simulink model "power_KundurTwoAreaSystem"  (R2021b)
settings: Solver=VariableStepAuto  StartTime=0.0  StopTime=20  MaxStep=1/60  RelTol=1e-4
PreLoadFcn:
  | Ts=50e-6;
  | Tctrl=2*Ts;
  | PSSMODEL=1;
model workspace (MAT data in the model file):
  LOL = 0
undefined symbols (not defined in the file or in its folder): D1, Delta
libraries: spsGenericPowerSystemStabilizerLib x8, spsThreePhaseVIMeasurementLib x6, spsLoadFlowBusLib x6, spsThreePhaseParallelRLCLoadLib x4, spsThreePhasePISectionLineLib x4, spsSynchronousMachinepuStandardLib x4, spsExcitationSystemLib x4, spsSteamTurbineandGovernorLib x4, spsThreePhaseSeriesRLCLoadLib x4, spsThreePhaseTransformerTwoWindingsLib x4, spsThreePhaseBreakerLib x2, spsDistributedParametersLineLib x2
(part 2 of 2)

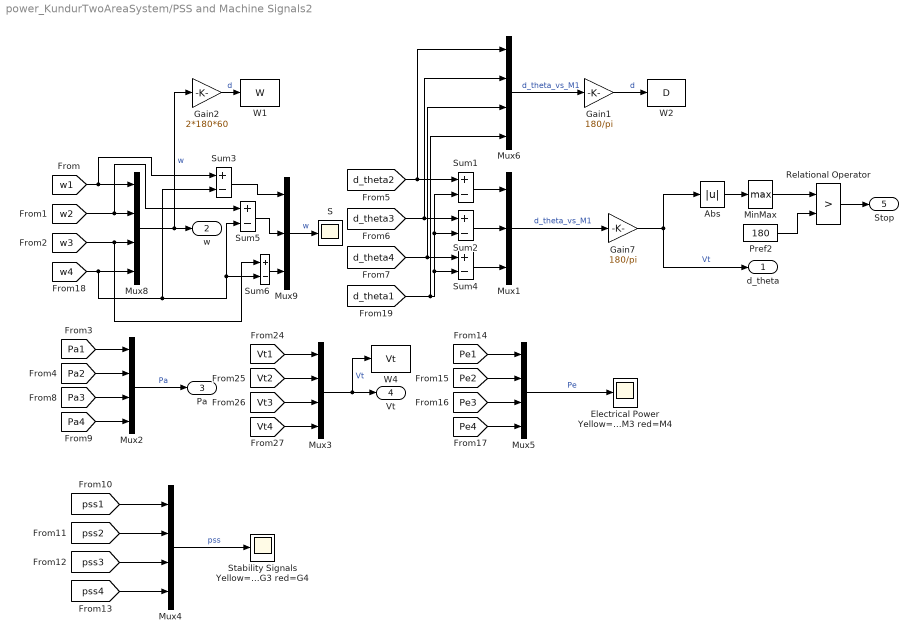
== system power_KundurTwoAreaSystem/PSS and Machine Signals2 ==
  Abs : Abs  SaturateOnIntegerOverflow=on
  "Electrical Power Yellow=M1 mag=M2 cyan=M3 red=M4 " : Scope
  Gain1 : Gain  Gain=180/pi
  Gain2 : Gain  Gain=2*180*60
  Gain7 : Gain  Gain=180/pi
  MinMax : MinMax  Function=max  InputSameDT=on  SaturateOnIntegerOverflow=on
  Mux1 : Mux  Inputs=3
  Mux{2..6,8} (6 alike) : Mux
  Mux9 : Mux  Inputs=3
  Pref2 : Constant  Value=180
  Relational Operator : RelationalOperator  Operator=>  RndMeth=Nearest  InputSameDT=on
  S : Scope
  "Stability Signals Yellow=G1 mag=G2 cyan=G3 red=G4 " : Scope
  Sum{1..6} (6 alike) : Sum  Inputs=+-  InputSameDT=on  SaturateOnIntegerOverflow=on  OutDataTypeStr=Inherit: Same as first input
  W1 : ToWorkspace  VariableName=W  SampleTime=-1
  W2 : ToWorkspace  VariableName=D  SampleTime=-1
  W4 : ToWorkspace  VariableName=Vt  SampleTime=-1
  d_theta : Outport  VectorParamsAs1DForOutWhenUnconnected=off
  w : Outport  Port=2  VectorParamsAs1DForOutWhenUnconnected=off
  Pa : Outport  Port=3  VectorParamsAs1DForOutWhenUnconnected=off
  Vt : Outport  Port=4  VectorParamsAs1DForOutWhenUnconnected=off
  Stop : Outport  Port=5  VectorParamsAs1DForOutWhenUnconnected=off
  wires:
  [Pa1] -> Mux2/1
  Mux4/1 -> "Stability Signals Yellow=G1 mag=G2 cyan=G3 red=G4 "/1  "pss"
  [pss1] -> Mux4/1
  [pss2] -> Mux4/2
  [pss4] -> Mux4/4
  [pss3] -> Mux4/3
  Mux8/1 -> Gain2/1, w/1  "w"
  Relational Operator/1 -> Stop/1
  Mux2/1 -> Pa/1  "Pa"
  [Pa2] -> Mux2/2
  [Pa3] -> Mux2/3
  [Pa4] -> Mux2/4
  [Vt1] -> Mux3/1
  [Vt2] -> Mux3/2
  [Vt3] -> Mux3/3
  [Vt4] -> Mux3/4
  Mux3/1 -> Vt/1, W4/1  "Vt"
  [Pe1] -> Mux5/1
  [Pe2] -> Mux5/2
  [Pe3] -> Mux5/3
  [Pe4] -> Mux5/4
  Mux5/1 -> "Electrical Power Yellow=M1 mag=M2 cyan=M3 red=M4 "/1  "Pe"
  [w1] -> Mux8/1, Sum3/1
  [w2] -> Mux8/2, Sum5/1
  [w3] -> Mux8/3, Sum6/1
  [w4] -> Mux8/4, Sum3/2, Sum6/2, Sum5/2
  Sum3/1 -> Mux9/1
  Sum5/1 -> Mux9/2
  Sum6/1 -> Mux9/3
  Mux1/1 -> Gain7/1  "d_theta_vs_M1"
  Abs/1 -> MinMax/1
  Pref2/1 -> Relational Operator/2
  MinMax/1 -> Relational Operator/1
  [d_theta2] -> Mux6/1, Sum1/1
  Sum1/1 -> Mux1/1
  [d_theta3] -> Mux6/2, Sum2/1
  [d_theta4] -> Mux6/3, Sum4/1
  [d_theta1] -> Mux6/4, Sum4/2, Sum2/2, Sum1/2
  Sum2/1 -> Mux1/2
  Sum4/1 -> Mux1/3
  Mux9/1 -> S/1  "w"
  Gain7/1 -> d_theta/1, Abs/1  "Vt"
  Mux6/1 -> Gain1/1  "d_theta_vs_M1"
  Gain1/1 -> W2/1  "d"
  Gain2/1 -> W1/1  "d"

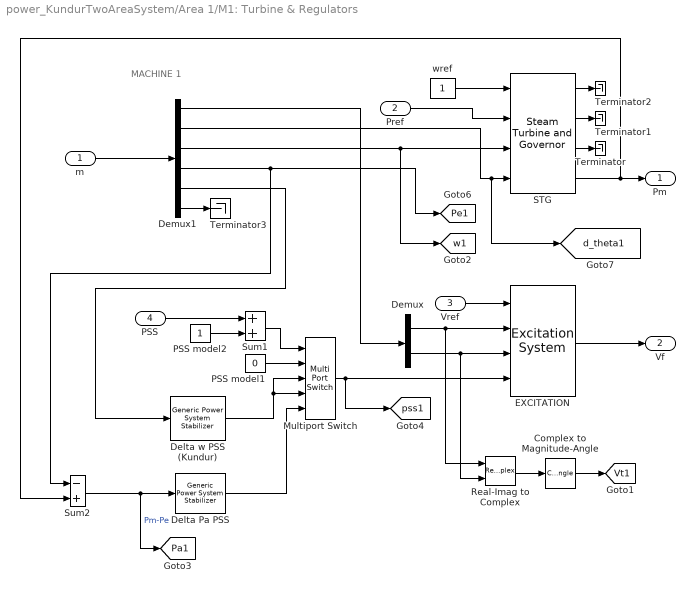
== system power_KundurTwoAreaSystem/Area 1/M1: Turbine & Regulators ==
  note: MACHINE 1
  m : Inport
  Pref : Inport  Port=2
  Vref : Inport  Port=3
  PSS : Inport  Port=4
  Complex to Magnitude-Angle : ComplexToMagnitudeAngle  Output=Magnitude
  Delta Pa PSS : spsGenericPowerSystemStabilizerLib/Generic Power System Stabilizer  Tsensor=15e-3  K=2.5*1.25  Twashout=1  Tleadlag1=[60e-3 1]  Tleadlag2=[0 0]  VSlimits=[-0.15 0.15]  Vinit=0  Plot_On=off  MagdB_On=on  FreqRange=logspace(-2,2,500)
      settings: SourceProductBaseCode=PS
  Delta w PSS (Kundur) : spsGenericPowerSystemStabilizerLib/Generic Power System Stabilizer  Tsensor=15e-3  K=30  Twashout=10  Tleadlag1=[50e-3 20e-3]  Tleadlag2=[3 5.4]  VSlimits=[-0.15 0.15]  Vinit=0  Plot_On=off  MagdB_On=on  FreqRange=logspace(-2,2,500)
      settings: SourceProductBaseCode=PS
  Demux : Demux  Outputs=2
      settings: DisplayOption=none
  Demux1 : Demux  Outputs=[2 1 1 1 1 1]
  EXCITATION : spsExcitationSystemLib/Excitation System  tr=20e-3  reg=[ 200, 0.001 ]  exc=[ 1, 0 ]  tgr=[ 0, 0 ]  damp=[ 0, 0 ]  sat=[ 0, 0 ]  lim=[-12.3 , 12.3, 0 ]  v0=[1,1.83395]
      settings: SourceProductBaseCode=PS
  Multiport Switch : MultiPortSwitch  Inputs=4  InputSameDT=on
  PSS model1 : Constant  Value=0
  PSS model2 : Constant
  Real-Imag to Complex : RealImagToComplex
  STG : spsSteamTurbineandGovernorLib/Steam Turbine and Governor  gentype=Tandem-compound (single mass)  reg1="[ 1  0.05    0 ]"  reg2="[ 0.001  0.15 ]"  reg3="[ -0.1  0.1  0  4.496 ]"  N=3600  turb1="[ 0  10   3.3   0.5   ]"  turb2="[   0   0.36    0.36   0.28   ]"  HA="[ 0.046  1.430  1.465   0.192 ]"  KA="[ 90.44  53.88  64.59   62.94  ]"  DA="[ 0.0115  0.3575  0.3663   0.0137  ]"  ini1=0.7778  ini2=[0.779316,-31.4247]
      settings: SourceProductBaseCode=PS
  Sum1 : Sum  InputSameDT=on  SaturateOnIntegerOverflow=on  OutDataTypeStr=Inherit: Same as first input
  Sum2 : Sum  Inputs=-+  InputSameDT=on  SaturateOnIntegerOverflow=on  OutDataTypeStr=Inherit: Same as first input
  Terminator{,1..3} (4 alike) : Terminator
  wref : Constant
  Pm : Outport  InitialOutput=0  VectorParamsAs1DForOutWhenUnconnected=off
  Vf : Outport  Port=2  InitialOutput=0  VectorParamsAs1DForOutWhenUnconnected=off
  tag scope: Pa1=global, Pe1=global, Vt1=global, d_theta1=global, pss1=global, w1=global
  wires:
  Demux/1 -> Real-Imag to Complex/1, EXCITATION/2
  Demux/2 -> Real-Imag to Complex/2, EXCITATION/3
  wref/1 -> STG/1
  Pref/1 -> STG/2
  m/1 -> Demux1/1
  Vref/1 -> EXCITATION/1
  Real-Imag to Complex/1 -> Complex to Magnitude-Angle/1
  EXCITATION/1 -> Vf/1
  Complex to Magnitude-Angle/1 -> [Vt1]
  Demux1/6 -> Terminator3/1
  PSS model1/1 -> Multiport Switch/2
  Delta w PSS (Kundur)/1 -> Multiport Switch/4, Multiport Switch/3
  Delta Pa PSS/1 -> Multiport Switch/5
  PSS model2/1 -> Sum1/2
  Sum1/1 -> Multiport Switch/1
  PSS/1 -> Sum1/1
  Demux1/1 -> Demux/1
  Demux1/3 -> [w1], STG/3
  Demux1/4 -> Sum2/1, [Pe1]
  Demux1/5 -> Delta w PSS (Kundur)/1
  Sum2/1 -> Delta Pa PSS/1, [Pa1]  "Pm-Pe"
  STG/3 -> Terminator/1
  Demux1/2 -> [d_theta1], STG/4
  STG/4 -> Pm/1, Sum2/2
  STG/2 -> Terminator1/1
  STG/1 -> Terminator2/1
  Multiport Switch/1 -> EXCITATION/4, [pss1]

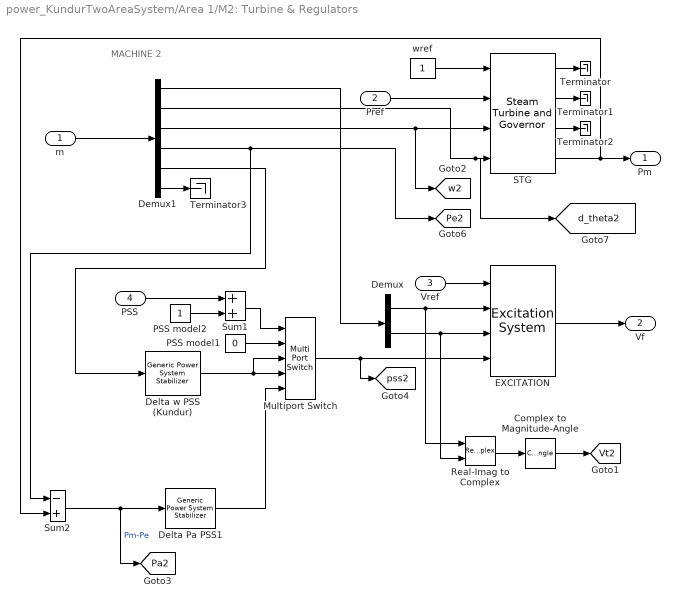
== system power_KundurTwoAreaSystem/Area 1/M2: Turbine & Regulators ==
  note: MACHINE 2
  m : Inport
  Pref : Inport  Port=2
  Vref : Inport  Port=3
  PSS : Inport  Port=4
  Complex to Magnitude-Angle : ComplexToMagnitudeAngle  Output=Magnitude
  Delta Pa PSS1 : spsGenericPowerSystemStabilizerLib/Generic Power System Stabilizer  Tsensor=15e-3  K=2.5*1.25  Twashout=1  Tleadlag1=[60e-3 1]  Tleadlag2=[0 0]  VSlimits=[-0.15 0.15]  Vinit=0  Plot_On=off  MagdB_On=on  FreqRange=logspace(-2,2,500)
      settings: SourceProductBaseCode=PS
  Delta w PSS (Kundur) : spsGenericPowerSystemStabilizerLib/Generic Power System Stabilizer  Tsensor=15e-3  K=30  Twashout=10  Tleadlag1=[50e-3 20e-3]  Tleadlag2=[3 5.4]  VSlimits=[-0.15 0.15]  Vinit=0  Plot_On=off  MagdB_On=on  FreqRange=logspace(-2,2,500)
      settings: SourceProductBaseCode=PS
  Demux : Demux  Outputs=2
      settings: DisplayOption=none
  Demux1 : Demux  Outputs=[2 1 1 1 1 1]
  EXCITATION : spsExcitationSystemLib/Excitation System  tr=20e-3  reg=[ 200, 0.001 ]  exc=[ 1, 0 ]  tgr=[ 0, 0 ]  damp=[ 0, 0 ]  sat=[ 0, 0 ]  lim=[ -12 , 12, 0 ]  v0=[1,1.83395]
      settings: SourceProductBaseCode=PS
  Multiport Switch : MultiPortSwitch  Inputs=4  InputSameDT=on
  PSS model1 : Constant  Value=0
  PSS model2 : Constant
  Real-Imag to Complex : RealImagToComplex
  STG : spsSteamTurbineandGovernorLib/Steam Turbine and Governor  gentype=Tandem-compound (single mass)  reg1="[ 1  0.05    0 ]"  reg2="[ 0.001  0.15 ]"  reg3="[ -0.1  0.1  0  4.496 ]"  N=3600  turb1="[ 0  10   3.3   0.5   ]"  turb2="[   0   0.36    0.36   0.28   ]"  HA="[ 0.046  1.430  1.465   0.192 ]"  KA="[ 90.44  53.88  64.59   62.94  ]"  DA="[ 0.0115  0.3575  0.3663   0.0137  ]"  ini1=0.7777  ini2=[0.779243,-42.8075]
      settings: SourceProductBaseCode=PS
  Sum1 : Sum  InputSameDT=on  SaturateOnIntegerOverflow=on  OutDataTypeStr=Inherit: Same as first input
  Sum2 : Sum  Inputs=-+  InputSameDT=on  SaturateOnIntegerOverflow=on  OutDataTypeStr=Inherit: Same as first input
  Terminator{,1..3} (4 alike) : Terminator
  wref : Constant
  Pm : Outport  InitialOutput=0  VectorParamsAs1DForOutWhenUnconnected=off
  Vf : Outport  Port=2  InitialOutput=0  VectorParamsAs1DForOutWhenUnconnected=off
  tag scope: Pa2=global, Pe2=global, Vt2=global, d_theta2=global, pss2=global, w2=global
  wires:
  Sum2/1 -> Delta Pa PSS1/1, [Pa2]  "Pm-Pe"
  Demux1/5 -> Delta w PSS (Kundur)/1
  Demux1/4 -> Sum2/1, [Pe2]
  Demux1/3 -> [w2], STG/3
  Demux1/1 -> Demux/1
  PSS/1 -> Sum1/1
  Sum1/1 -> Multiport Switch/1
  PSS model2/1 -> Sum1/2
  Delta Pa PSS1/1 -> Multiport Switch/5
  Delta w PSS (Kundur)/1 -> Multiport Switch/4, Multiport Switch/3
  PSS model1/1 -> Multiport Switch/2
  Multiport Switch/1 -> [pss2], EXCITATION/4
  Demux1/6 -> Terminator3/1
  Complex to Magnitude-Angle/1 -> [Vt2]
  EXCITATION/1 -> Vf/1
  Real-Imag to Complex/1 -> Complex to Magnitude-Angle/1
  Vref/1 -> EXCITATION/1
  Pref/1 -> STG/2
  wref/1 -> STG/1
  Demux/2 -> Real-Imag to Complex/2, EXCITATION/3
  Demux/1 -> Real-Imag to Complex/1, EXCITATION/2
  STG/1 -> Terminator/1
  STG/2 -> Terminator1/1
  STG/3 -> Terminator2/1
  STG/4 -> Pm/1, Sum2/2
  Demux1/2 -> [d_theta2], STG/4
  m/1 -> Demux1/1

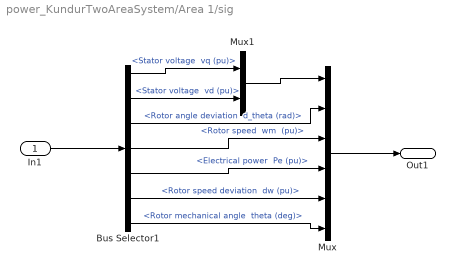
== system power_KundurTwoAreaSystem/Area 1/sig ==
  In1 : Inport
  Bus Selector1 : BusSelector  OutputSignals="dq0 components.Stator voltage  vq (pu),dq0 components.Stator voltage  vd (pu),Mechanical.Rotor angle deviation  d_theta (rad),Mechanical.Rotor speed  wm  (pu),Mechanical.Electrical power  Pe (pu),Mechanical.Rotor speed deviation  dw (pu),Mechanical.Rotor mechanical angle  theta (deg)"
  Mux : Mux  Inputs=6
  Mux1 : Mux  Inputs=2
  Out1 : Outport  VectorParamsAs1DForOutWhenUnconnected=off
  wires:
  Mux/1 -> Out1/1
  In1/1 -> Bus Selector1/1
  Bus Selector1/7 -> Mux/6  "<Rotor mechanical angle  theta (deg)>"
  Bus Selector1/6 -> Mux/5  "<Rotor speed deviation  dw (pu)>"
  Bus Selector1/5 -> Mux/4  "<Electrical power  Pe (pu)>"
  Bus Selector1/4 -> Mux/3  "<Rotor speed  wm  (pu)>"
  Bus Selector1/3 -> Mux/2  "<Rotor angle deviation  d_theta (rad)>"
  Bus Selector1/2 -> Mux1/2  "<Stator voltage  vd (pu)>"
  Bus Selector1/1 -> Mux1/1  "<Stator voltage  vq (pu)>"
  Mux1/1 -> Mux/1

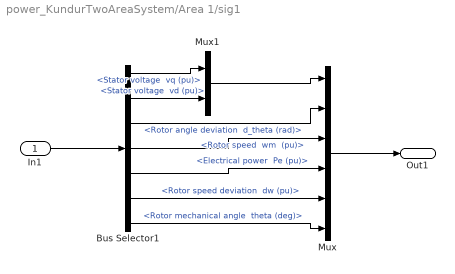
== system power_KundurTwoAreaSystem/Area 1/sig1 ==
  In1 : Inport
  Bus Selector1 : BusSelector  OutputSignals="dq0 components.Stator voltage  vq (pu),dq0 components.Stator voltage  vd (pu),Mechanical.Rotor angle deviation  d_theta (rad),Mechanical.Rotor speed  wm  (pu),Mechanical.Electrical power  Pe (pu),Mechanical.Rotor speed deviation  dw (pu),Mechanical.Rotor mechanical angle  theta (deg)"
  Mux : Mux  Inputs=6
  Mux1 : Mux  Inputs=2
  Out1 : Outport  VectorParamsAs1DForOutWhenUnconnected=off
  wires:
  Mux1/1 -> Mux/1
  Bus Selector1/1 -> Mux1/1  "<Stator voltage  vq (pu)>"
  Bus Selector1/2 -> Mux1/2  "<Stator voltage  vd (pu)>"
  Bus Selector1/3 -> Mux/2  "<Rotor angle deviation  d_theta (rad)>"
  Bus Selector1/4 -> Mux/3  "<Rotor speed  wm  (pu)>"
  Bus Selector1/5 -> Mux/4  "<Electrical power  Pe (pu)>"
  Bus Selector1/6 -> Mux/5  "<Rotor speed deviation  dw (pu)>"
  Bus Selector1/7 -> Mux/6  "<Rotor mechanical angle  theta (deg)>"
  In1/1 -> Bus Selector1/1
  Mux/1 -> Out1/1

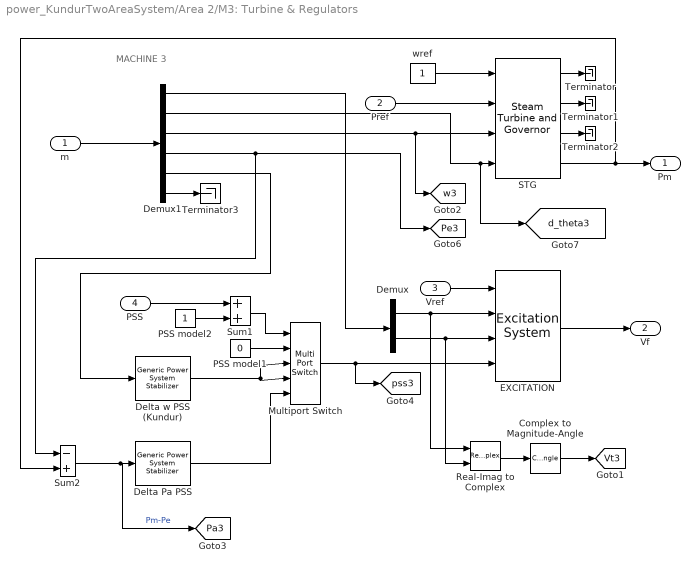
== system power_KundurTwoAreaSystem/Area 2/M3: Turbine & Regulators ==
  note: MACHINE 3
  m : Inport
  Pref : Inport  Port=2
  Vref : Inport  Port=3
  PSS : Inport  Port=4
  Complex to Magnitude-Angle : ComplexToMagnitudeAngle  Output=Magnitude
  Delta Pa PSS : spsGenericPowerSystemStabilizerLib/Generic Power System Stabilizer  Tsensor=15e-3  K=2.5*1.25  Twashout=1  Tleadlag1=[60e-3 1]  Tleadlag2=[0 0]  VSlimits=[-0.15 0.15]  Vinit=0  Plot_On=off  MagdB_On=on  FreqRange=logspace(-2,2,500)
      settings: SourceProductBaseCode=PS
  Delta w PSS (Kundur) : spsGenericPowerSystemStabilizerLib/Generic Power System Stabilizer  Tsensor=15e-3  K=30  Twashout=10  Tleadlag1=[50e-3 20e-3]  Tleadlag2=[3 5.4]  VSlimits=[-0.15 0.15]  Vinit=0  Plot_On=off  MagdB_On=on  FreqRange=logspace(-2,2,500)
      settings: SourceProductBaseCode=PS
  Demux : Demux  Outputs=2
      settings: DisplayOption=none
  Demux1 : Demux  Outputs=[2 1 1 1 1 1]
  EXCITATION : spsExcitationSystemLib/Excitation System  tr=20e-3  reg=[ 200, 0.001 ]  exc=[ 1, 0 ]  tgr=[ 0, 0 ]  damp=[ 0, 0 ]  sat=[ 0, 0 ]  lim=[ -12.3 , 12.3, 0 ]  v0=[1,1.83395]
      settings: SourceProductBaseCode=PS
  Multiport Switch : MultiPortSwitch  Inputs=4  InputSameDT=on
  PSS model1 : Constant  Value=0
  PSS model2 : Constant
  Real-Imag to Complex : RealImagToComplex
  STG : spsSteamTurbineandGovernorLib/Steam Turbine and Governor  gentype=Tandem-compound (single mass)  reg1="[ 1  0.05    0 ]"  reg2="[ 0.001  0.15 ]"  reg3="[ -0.1  0.1  0  4.496 ]"  N=3600  turb1="[ 0  10   3.3   0.5   ]"  turb2="[   0   0.36    0.36   0.28   ]"  HA="[ 0.046  1.430  1.465   0.192 ]"  KA="[ 90.44  53.88  64.59   62.94  ]"  DA="[ 0.0115  0.3575  0.3663   0.0137  ]"  ini1=0.798889  ini2=[0.800505,-56.3243]
      settings: SourceProductBaseCode=PS
  Sum1 : Sum  InputSameDT=on  SaturateOnIntegerOverflow=on  OutDataTypeStr=Inherit: Same as first input
  Sum2 : Sum  Inputs=-+  InputSameDT=on  SaturateOnIntegerOverflow=on  OutDataTypeStr=Inherit: Same as first input
  Terminator{,1..3} (4 alike) : Terminator
  wref : Constant
  Pm : Outport  InitialOutput=0  VectorParamsAs1DForOutWhenUnconnected=off
  Vf : Outport  Port=2  InitialOutput=0  VectorParamsAs1DForOutWhenUnconnected=off
  tag scope: Pa3=global, Pe3=global, Vt3=global, d_theta3=global, pss3=global, w3=global
  wires:
  Sum2/1 -> [Pa3], Delta Pa PSS/1  "Pm-Pe"
  Demux1/5 -> Delta w PSS (Kundur)/1
  Demux1/4 -> Sum2/1, [Pe3]
  Demux1/3 -> [w3], STG/3
  Demux1/1 -> Demux/1
  PSS/1 -> Sum1/1
  Sum1/1 -> Multiport Switch/1
  PSS model2/1 -> Sum1/2
  Delta Pa PSS/1 -> Multiport Switch/5
  Delta w PSS (Kundur)/1 -> Multiport Switch/4, Multiport Switch/3
  PSS model1/1 -> Multiport Switch/2
  Multiport Switch/1 -> [pss3], EXCITATION/4
  Demux1/6 -> Terminator3/1
  Complex to Magnitude-Angle/1 -> [Vt3]
  EXCITATION/1 -> Vf/1
  Real-Imag to Complex/1 -> Complex to Magnitude-Angle/1
  Vref/1 -> EXCITATION/1
  m/1 -> Demux1/1
  Pref/1 -> STG/2
  wref/1 -> STG/1
  Demux/2 -> Real-Imag to Complex/2, EXCITATION/3
  Demux/1 -> Real-Imag to Complex/1, EXCITATION/2
  Demux1/2 -> [d_theta3], STG/4
  STG/1 -> Terminator/1
  STG/2 -> Terminator1/1
  STG/3 -> Terminator2/1
  STG/4 -> Pm/1, Sum2/2

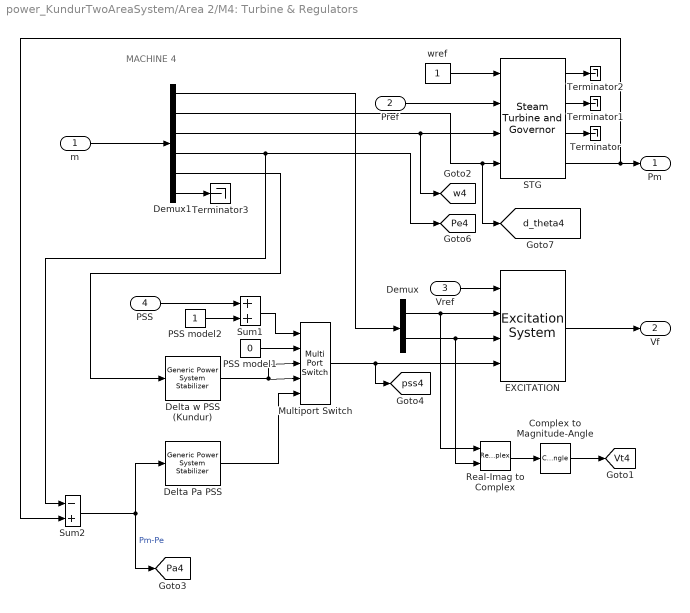
== system power_KundurTwoAreaSystem/Area 2/M4: Turbine & Regulators ==
  note: MACHINE 4
  m : Inport
  Pref : Inport  Port=2
  Vref : Inport  Port=3
  PSS : Inport  Port=4
  Complex to Magnitude-Angle : ComplexToMagnitudeAngle  Output=Magnitude
  "Delta Pa PSS " : spsGenericPowerSystemStabilizerLib/Generic Power System Stabilizer  Tsensor=15e-3  K=2.5*1.25  Twashout=1  Tleadlag1=[60e-3 1]  Tleadlag2=[0 0]  VSlimits=[-0.15 0.15]  Vinit=0  Plot_On=off  MagdB_On=on  FreqRange=logspace(-2,2,500)
      settings: SourceProductBaseCode=PS
  Delta w PSS (Kundur) : spsGenericPowerSystemStabilizerLib/Generic Power System Stabilizer  Tsensor=15e-3  K=30  Twashout=10  Tleadlag1=[50e-3 20e-3]  Tleadlag2=[3 5.4]  VSlimits=[-0.15 0.15]  Vinit=0  Plot_On=off  MagdB_On=on  FreqRange=logspace(-2,2,500)
      settings: SourceProductBaseCode=PS
  Demux : Demux  Outputs=2
      settings: DisplayOption=none
  Demux1 : Demux  Outputs=[2 1 1 1 1 1]
  EXCITATION : spsExcitationSystemLib/Excitation System  tr=20e-3  reg=[ 200, 0.001 ]  exc=[ 1, 0 ]  tgr=[ 0, 0 ]  damp=[ 0, 0 ]  sat=[ 0, 0 ]  lim=[ -12.3 , 12.3, 0 ]  v0=[1,1.83395]
      settings: SourceProductBaseCode=PS
  Multiport Switch : MultiPortSwitch  Inputs=4  InputSameDT=on
  PSS model1 : Constant  Value=0
  PSS model2 : Constant
  Real-Imag to Complex : RealImagToComplex
  STG : spsSteamTurbineandGovernorLib/Steam Turbine and Governor  gentype=Tandem-compound (single mass)  reg1="[ 1  0.05    0 ]"  reg2="[ 0.001  0.15 ]"  reg3="[ -0.1  0.1  0  4.496 ]"  N=3600  turb1="[ 0  10   3.3   0.5   ]"  turb2="[   0   0.36    0.36   0.28   ]"  HA="[ 0.046  1.430  1.465   0.192 ]"  KA="[ 90.44  53.88  64.59   62.94  ]"  DA="[ 0.0115  0.3575  0.3663   0.0137  ]"  ini1=0.7778  ini2=[0.779311,-67.7513]
      settings: SourceProductBaseCode=PS
  Sum1 : Sum  InputSameDT=on  SaturateOnIntegerOverflow=on  OutDataTypeStr=Inherit: Same as first input
  Sum2 : Sum  Inputs=-+  InputSameDT=on  SaturateOnIntegerOverflow=on  OutDataTypeStr=Inherit: Same as first input
  Terminator{,1..3} (4 alike) : Terminator
  wref : Constant
  Pm : Outport  InitialOutput=0  VectorParamsAs1DForOutWhenUnconnected=off
  Vf : Outport  Port=2  InitialOutput=0  VectorParamsAs1DForOutWhenUnconnected=off
  tag scope: Pa4=global, Pe4=global, Vt4=global, d_theta4=global, pss4=global, w4=global
  wires:
  Demux/1 -> Real-Imag to Complex/1, EXCITATION/2
  Demux/2 -> Real-Imag to Complex/2, EXCITATION/3
  STG/4 -> Pm/1, Sum2/2
  wref/1 -> STG/1
  Pref/1 -> STG/2
  m/1 -> Demux1/1
  Vref/1 -> EXCITATION/1
  STG/3 -> Terminator/1
  Real-Imag to Complex/1 -> Complex to Magnitude-Angle/1
  EXCITATION/1 -> Vf/1
  Complex to Magnitude-Angle/1 -> [Vt4]
  Demux1/6 -> Terminator3/1
  Multiport Switch/1 -> EXCITATION/4, [pss4]
  PSS model1/1 -> Multiport Switch/2
  Delta w PSS (Kundur)/1 -> Multiport Switch/4, Multiport Switch/3
  "Delta Pa PSS "/1 -> Multiport Switch/5
  PSS model2/1 -> Sum1/2
  Sum1/1 -> Multiport Switch/1
  PSS/1 -> Sum1/1
  Demux1/1 -> Demux/1
  Demux1/3 -> [w4], STG/3
  Demux1/4 -> Sum2/1, [Pe4]
  Demux1/5 -> Delta w PSS (Kundur)/1
  Sum2/1 -> "Delta Pa PSS "/1, [Pa4]  "Pm-Pe"
  STG/2 -> Terminator1/1
  STG/1 -> Terminator2/1
  Demux1/2 -> [d_theta4], STG/4

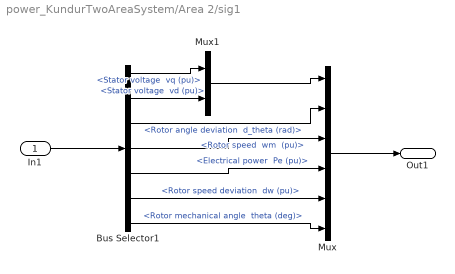
== system power_KundurTwoAreaSystem/Area 2/sig1 ==
  In1 : Inport
  Bus Selector1 : BusSelector  OutputSignals="dq0 components.Stator voltage  vq (pu),dq0 components.Stator voltage  vd (pu),Mechanical.Rotor angle deviation  d_theta (rad),Mechanical.Rotor speed  wm  (pu),Mechanical.Electrical power  Pe (pu),Mechanical.Rotor speed deviation  dw (pu),Mechanical.Rotor mechanical angle  theta (deg)"
  Mux : Mux  Inputs=6
  Mux1 : Mux  Inputs=2
  Out1 : Outport  VectorParamsAs1DForOutWhenUnconnected=off
  wires:
  Mux1/1 -> Mux/1
  Bus Selector1/1 -> Mux1/1  "<Stator voltage  vq (pu)>"
  Bus Selector1/2 -> Mux1/2  "<Stator voltage  vd (pu)>"
  Bus Selector1/3 -> Mux/2  "<Rotor angle deviation  d_theta (rad)>"
  Bus Selector1/4 -> Mux/3  "<Rotor speed  wm  (pu)>"
  Bus Selector1/5 -> Mux/4  "<Electrical power  Pe (pu)>"
  Bus Selector1/6 -> Mux/5  "<Rotor speed deviation  dw (pu)>"
  Bus Selector1/7 -> Mux/6  "<Rotor mechanical angle  theta (deg)>"
  In1/1 -> Bus Selector1/1
  Mux/1 -> Out1/1

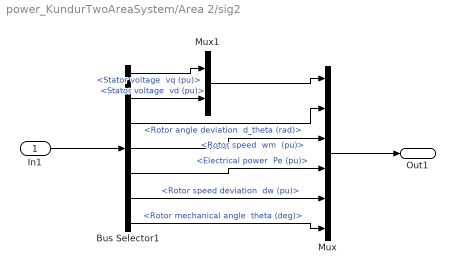
== system power_KundurTwoAreaSystem/Area 2/sig2 ==
  In1 : Inport
  Bus Selector1 : BusSelector  OutputSignals="dq0 components.Stator voltage  vq (pu),dq0 components.Stator voltage  vd (pu),Mechanical.Rotor angle deviation  d_theta (rad),Mechanical.Rotor speed  wm  (pu),Mechanical.Electrical power  Pe (pu),Mechanical.Rotor speed deviation  dw (pu),Mechanical.Rotor mechanical angle  theta (deg)"
  Mux : Mux  Inputs=6
  Mux1 : Mux  Inputs=2
  Out1 : Outport  VectorParamsAs1DForOutWhenUnconnected=off
  wires:
  Mux1/1 -> Mux/1
  Bus Selector1/1 -> Mux1/1  "<Stator voltage  vq (pu)>"
  Bus Selector1/2 -> Mux1/2  "<Stator voltage  vd (pu)>"
  Bus Selector1/3 -> Mux/2  "<Rotor angle deviation  d_theta (rad)>"
  Bus Selector1/4 -> Mux/3  "<Rotor speed  wm  (pu)>"
  Bus Selector1/5 -> Mux/4  "<Electrical power  Pe (pu)>"
  Bus Selector1/6 -> Mux/5  "<Rotor speed deviation  dw (pu)>"
  Bus Selector1/7 -> Mux/6  "<Rotor mechanical angle  theta (deg)>"
  In1/1 -> Bus Selector1/1
  Mux/1 -> Out1/1
